simulink model "MobileBaseControl"  (R2022a)
settings: Solver=FixedStepDiscrete  StartTime=0.0  StopTime=10.0  RelTol=1e-3
settings Model: Creator=EarthPhisek  LastModifiedBy=EarthPhisek
settings OptimizationCC: EnhancedBackFolding=on  PassReuseOutputArgsAs=Individual arguments  ZeroExternalMemoryAtStartup=off  ZeroInternalMemoryAtStartup=off  MaxStackSize=64  OptimizeBlockOrder=speed  DifferentSizesBufferReuse=on  OptimizationCustomize=off  EfficientTunableParamExpr=on
settings DebuggingCC: ParameterTunabilityLossMsg=error
settings HardwareCC: UseEmbeddedCoderFeatures=off
settings SFSimCC: MATLABDynamicMemAlloc=off
settings RTWCC: SystemTargetFile=ert.tlc  HardwareBoard=Robot Operating System 2 (ROS 2)  TLCOptions="-aInlineSetEventsForThisBaseRateFcn=TLC_FALSE -aSuppressMultiTaskScheduler=TLC_FALSE  -aRateBasedStepFcn=0"  TemplateMakefile=ert_default_tmf  Toolchain=Colcon Tools  TargetLang=C++
settings CodeAppCC: ForceParamTrailComments=on  IgnoreCustomStorageClasses=off  OperatorAnnotations=on  SimulinkDataObjDesc=on  SFDataObjDesc=on  InsertBlockDesc=on
settings ERTTargetCC: CodeInterfacePackaging=C++ class  SupportNonInlinedSFcns=on  RootIOFormat=Structure reference

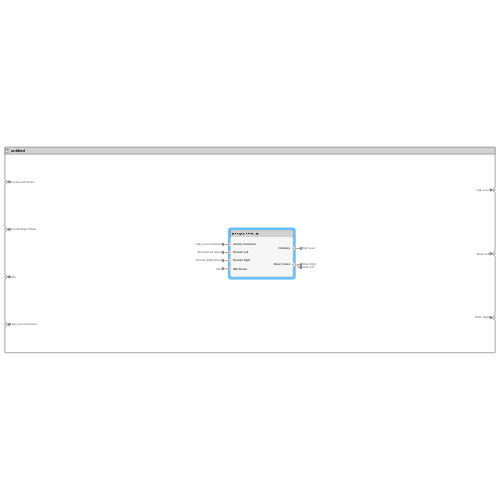
[thumbnail: Simulink's stored preview of the top-level diagram]
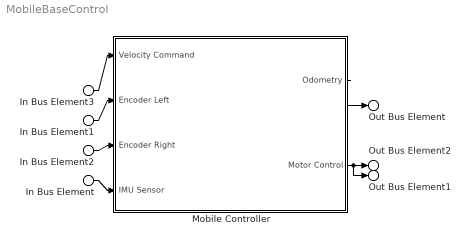
== system MobileBaseControl ==
  In Bus Element1 : Inport  PortName=Encoder Left Wheel
  In Bus Element2 : Inport  Port=2  PortName=Encoder Right Wheel
  In Bus Element : Inport  Port=3  PortName=IMU
  In Bus Element3 : Inport  Port=4  PortName=High Level Command
  Mobile Controller : Subsystem
      settings: PortSchema="{\"entries\":[{\"content\":{\"headerSize\":26,\"margin\":15,\"minimumSpacing\":25,\"sides\":[{\"content\":{\"connectorIds\":[\"In1\",\"In2\",\"In3\",\"In4\"]},\"type\":\"ConnectorPlacement.EquallySpacedRectSide\",\"uuid\":\"dd41dd12-49ec-4c74-984d-ae398e001f17\"},{\"content\":{\"connectorIds\":[\"Out1\",\"Out2\"],\"side\":\"RIGHT\"},\"type\":\"ConnectorPlacement.EquallySpacedRectSide\",\"uuid\":\"7b6711d5-260d-4adb-8390-dd0a2fe64eed\"},{\"content\":{\"connectorIds\":[],\"side\":\"TOP\"},\"type\":\"ConnectorPlacement.EquallySpacedRectSide\",\"uuid\":\"51c2854e-5efe-4dec-8c07-70731026f3e8\"}]},\"type\":\"ConnectorPlacement.EquallySpacedConnector\",\"uuid\":\"aa3377b9-5458-4828-a095-24c10dd42ea0\"}],\"packageUris\":[\"http://schema.mathworks.com/mf0/Connector/R2020b\"],\"version\":\"1.0\"}"
  Out Bus Element : Outport  PortName=High Level
  Out Bus Element1 : Outport  Port=2  PortName=Motor Left
  Out Bus Element2 : Outport  Port=3  PortName=Motor Right
  wires:
  In Bus Element/1 -> Mobile Controller/4(IMU Sensor)
  In Bus Element1/1 -> Mobile Controller/2(Encoder Left)
  In Bus Element2/1 -> Mobile Controller/3(Encoder Right)
  In Bus Element3/1 -> Mobile Controller/1(Velocity Command)
  Mobile Controller/1(Odometry) -> Out Bus Element/1
  Mobile Controller/2(Motor Control) -> Out Bus Element2/1, Out Bus Element1/1

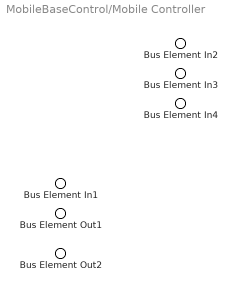
== system MobileBaseControl/Mobile Controller ==
  Bus Element In4 : Inport  PortName=Velocity Command
  Bus Element In2 : Inport  Port=2  PortName=Encoder Left
  Bus Element In3 : Inport  Port=3  PortName=Encoder Right
  Bus Element In1 : Inport  Port=4  PortName=IMU Sensor
  Bus Element Out1 : Outport  PortName=Odometry
  Bus Element Out2 : Outport  Port=2  PortName=Motor Control
